simulink model "state_feedback_torques"  (R2015b)
settings: Solver=VariableStepAuto  StartTime=0.0  StopTime=5  RelTol=1e-3
values from neighbouring files (symbols this model uses):
  A12 = A(1:3,4:6)    [StateSpace.m]
  Jx = 0.1    [Parameters.m]
  Jy = 0.1    [Parameters.m]
  Jz = 0.2    [Parameters.m]
  Lobs = (-place(A22',A12',[-60 -70 -80]))'    [StateSpace.m]
settings Model: Creator=USUARIO  LastModifiedBy=USUARIO

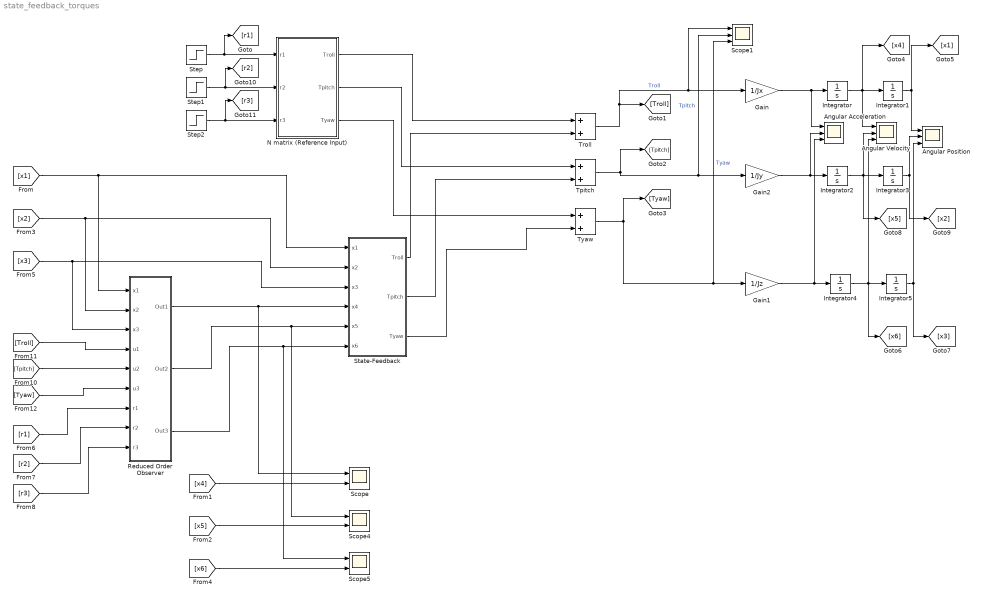
== system state_feedback_torques ==
  Angular Position : Scope  NumInputPorts=3
  Angular Velocity : Scope  NumInputPorts=3
  Angular Acceleration : Scope  NumInputPorts=3
  Gain : Gain  Gain=1/Jx
  Gain1 : Gain  Gain=1/Jz
  Gain2 : Gain  Gain=1/Jy
  Integrator{,1..5} (6 alike) : Integrator
  N matrix (Reference Input) : MATLAB Function  TreatAsAtomicUnit=on
  Reduced Order Observer : Subsystem
  Scope : Scope  NumInputPorts=2
  Scope1 : Scope  NumInputPorts=3
  Scope4 : Scope  NumInputPorts=2
  Scope5 : Scope  NumInputPorts=2
  "State-Feedback " : MATLAB Function  TreatAsAtomicUnit=on
  Step : Step  Time=0.2  After=0.5  SampleTime=0
  Step1 : Step  Time=0.2  After=0.3  SampleTime=0
  Step2 : Step  Time=0.2  After=0  SampleTime=0
  Tpitch : Sum
  Troll : Sum
  Tyaw : Sum
  wires:
  Gain/1 -> Angular Acceleration/1, Integrator/1
  Gain2/1 -> Angular Acceleration/2, Integrator2/1
  Gain1/1 -> Integrator4/1, Angular Acceleration/3
  Integrator4/1 -> Angular Velocity/3, [x6], Integrator5/1
  Integrator2/1 -> Angular Velocity/2, [x5], Integrator3/1
  Integrator/1 -> [x4], Angular Velocity/1, Integrator1/1
  Integrator1/1 -> Angular Position/1, [x1]
  Integrator3/1 -> Angular Position/2, [x2]
  Integrator5/1 -> Angular Position/3, [x3]
  "State-Feedback "/1(Troll) -> Troll/2
  "State-Feedback "/2(Tpitch) -> Tpitch/2
  "State-Feedback "/3(Tyaw) -> Tyaw/2
  [x1] -> "State-Feedback "/1(x1), Reduced Order Observer/1(x1)
  [x2] -> "State-Feedback "/2(x2), Reduced Order Observer/2(x2)
  [x3] -> "State-Feedback "/3(x3), Reduced Order Observer/3(x3)
  [Troll] -> Reduced Order Observer/4(u1)
  [Tpitch] -> Reduced Order Observer/5(u2)
  [Tyaw] -> Reduced Order Observer/6(u3)
  Reduced Order Observer/2(Out2) -> "State-Feedback "/5(x5), Scope4/1
  Reduced Order Observer/3(Out3) -> "State-Feedback "/6(x6), Scope5/1
  [x4] -> Scope/2
  [x5] -> Scope4/2
  [x6] -> Scope5/2
  Troll/1 -> Scope1/1, Gain/1, [Troll]  "Troll"
  Tyaw/1 -> Scope1/3, Gain1/1, [Tyaw]  "Tyaw"
  Tpitch/1 -> Scope1/2, Gain2/1, [Tpitch]  "Tpitch"
  Step2/1 -> [r3], N matrix (Reference Input)/3(r3)
  Step1/1 -> [r2], N matrix (Reference Input)/2(r2)
  Step/1 -> [r1], N matrix (Reference Input)/1(r1)
  [r1] -> Reduced Order Observer/7(r1)
  [r2] -> Reduced Order Observer/8(r2)
  [r3] -> Reduced Order Observer/9("r3 ")
  Reduced Order Observer/1(Out1) -> "State-Feedback "/4(x4), Scope/1
  N matrix (Reference Input)/1(Troll) -> Troll/1
  N matrix (Reference Input)/2(Tpitch) -> Tpitch/1
  N matrix (Reference Input)/3(Tyaw) -> Tyaw/1

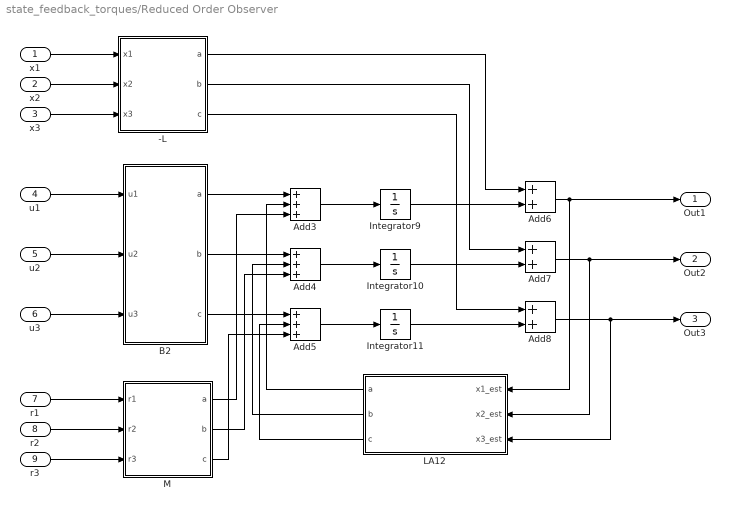
== system state_feedback_torques/Reduced Order Observer ==
  x1 : Inport
  x2 : Inport  Port=2
  x3 : Inport  Port=3
  u1 : Inport  Port=4
  u2 : Inport  Port=5
  u3 : Inport  Port=6
  r1 : Inport  Port=7
  r2 : Inport  Port=8
  "r3 " : Inport  Port=9
  "-L " : MATLAB Function  TreatAsAtomicUnit=on
  Add3 : Sum  Inputs=3
  Add4 : Sum  Inputs=3
  Add5 : Sum  Inputs=3
  Add6 : Sum  Inputs=2
  Add7 : Sum  Inputs=2
  Add8 : Sum  Inputs=2
  B2 : MATLAB Function  TreatAsAtomicUnit=on
  Integrator10 : Integrator
  Integrator11 : Integrator
  Integrator9 : Integrator
  LA12 : MATLAB Function  TreatAsAtomicUnit=on
  M : MATLAB Function  TreatAsAtomicUnit=on
  Out1 : Outport
  Out2 : Outport  Port=2
  Out3 : Outport  Port=3
  wires:
  Add4/1 -> Integrator10/1
  Add3/1 -> Integrator9/1
  Add5/1 -> Integrator11/1
  u2/1 -> B2/2(u2)
  B2/1(a) -> Add3/1
  B2/2(b) -> Add4/1
  B2/3(c) -> Add5/1
  LA12/1(a) -> Add3/2
  LA12/2(b) -> Add4/2
  LA12/3(c) -> Add5/2
  Add6/1 -> LA12/1(x1_est), Out1/1
  Add7/1 -> LA12/2(x2_est), Out2/1
  Add8/1 -> LA12/3(x3_est), Out3/1
  "-L "/3(c) -> Add8/1
  "-L "/1(a) -> Add6/1
  "-L "/2(b) -> Add7/1
  x2/1 -> "-L "/2(x2)
  x3/1 -> "-L "/3(x3)
  x1/1 -> "-L "/1(x1)
  Integrator9/1 -> Add6/2
  Integrator11/1 -> Add8/2
  Integrator10/1 -> Add7/2
  u1/1 -> B2/1(u1)
  u3/1 -> B2/3(u3)
  r2/1 -> M/2(r2)
  r1/1 -> M/1(r1)
  "r3 "/1 -> M/3(r3)
  M/1(a) -> Add3/3
  M/2(b) -> Add4/3
  M/3(c) -> Add5/3

== matlab function state_feedback_torques/State-Feedback  ==
  data: x1 input; Troll output; Tpitch output; Tyaw output; x2 input; x3 input; x4 input; x5 input; x6 input; F parameter
function [Troll,Tpitch,Tyaw]= F_matrix(x1, x2, x3, x4, x5, x6, F)
x=[x1;
    x2;
    x3;
    x4;
    x5;
    x6];

T=F*x;

Troll=T(1);
Tpitch=T(2);
Tyaw=T(3);

== matlab function state_feedback_torques/Reduced Order Observer/M ==
  data: r1 input; a output; b output; c output; r2 input; r3 input; M parameter
function [a,b,c] = M_matrix(r1, r2, r3, M)
r=[r1;
    r2;
    r3];

abc=M*r;

a=abc(1);
b=abc(2);
c=abc(3);

== matlab function state_feedback_torques/Reduced Order Observer/-L  ==
  data: x1 input; a output; b output; c output; x2 input; x3 input; Lobs parameter
function [a,b,c] = minusL_matrix(x1, x2, x3, Lobs)
x=[x1;
    x2;
    x3];

abc=-Lobs*x;

a=abc(1);
b=abc(2);
c=abc(3);

== matlab function state_feedback_torques/Reduced Order Observer/B2 ==
  data: u1 input; a output; b output; c output; u2 input; u3 input; B2 parameter
function [a, b, c] = B2_matrix(u1, u2, u3, B2)
u=[u1;
    u2;
    u3];

abc=B2*u;

a=abc(1);
b=abc(2);
c=abc(3);

== matlab function state_feedback_torques/Reduced Order Observer/LA12 ==
  data: x1_est input; x2_est input; x3_est input; a output; b output; c output; Lobs parameter; A12 parameter
function [a,b,c] = LA12_matrix(x1_est, x2_est, x3_est, Lobs, A12)
x=[x1_est;
    x2_est;
    x3_est];

abc=Lobs*A12*x;

a=abc(1);
b=abc(2);
c=abc(3);

== matlab function state_feedback_torques/N matrix (Reference Input) ==
  data: r1 input; Troll output; Tpitch output; Tyaw output; r2 input; r3 input; N parameter
function [Troll,Tpitch,Tyaw] = N_matrix(r1, r2, r3,N)
r=[r1;
    r2;
    r3];

T=N*r;

Troll=T(1);
Tpitch=T(2);
Tyaw=T(3);
